simulink model "MIMO"  (R2017a)
settings: Solver=VariableStepAuto  StartTime=0.0  StopTime=inf  RelTol=1e-3
InitFcn:
  | QPSK_ini
undefined symbols (not defined in the file or in its folder): oversampling_factor, rolloff_factor
libraries: commutil2 x4, commdigbbndpm3 x4, commfilt2 x4, commsync2 x4, commrandsrc3 x2, commchan3 x2, commrflib2 x2, dspsigops x2
settings Model: Creator=Arthur  LastModifiedBy=Arthur

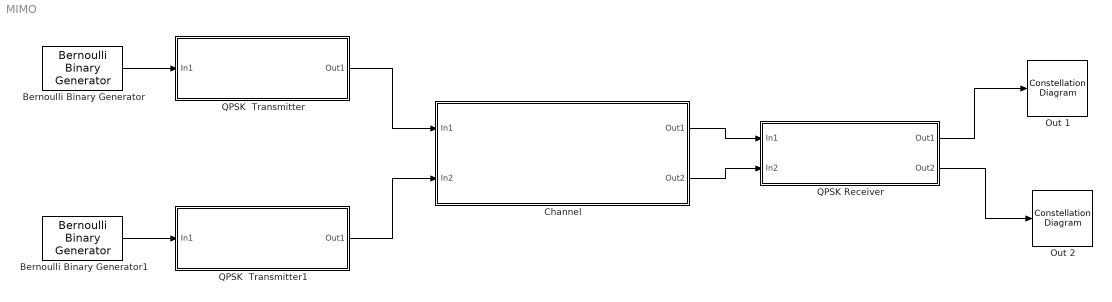
== system MIMO ==
  Bernoulli Binary Generator : commrandsrc3/Bernoulli Binary Generator  ProbabilityOfZero=0.5  SeedSource=Auto  Seed=0  SampleTime=1  SamplesPerFrame=512  OutputDataType=double  SimulateUsing=Interpreted execution
  Bernoulli Binary Generator1 : commrandsrc3/Bernoulli Binary Generator  ProbabilityOfZero=0.5  SeedSource=Auto  Seed=0  SampleTime=1  SamplesPerFrame=512  OutputDataType=double  SimulateUsing=Interpreted execution
  Channel : Subsystem
  Out 1 : ConstellationDiagram
  Out 2 : ConstellationDiagram
  QPSK  Transmitter : Subsystem
  QPSK  Transmitter1 : Subsystem
  QPSK Receiver : Subsystem
  wires:
  Bernoulli Binary Generator/1 -> QPSK  Transmitter/1(In1)
  Bernoulli Binary Generator1/1 -> QPSK  Transmitter1/1(In1)
  QPSK  Transmitter/1(Out1) -> Channel/1(In1)
  QPSK  Transmitter1/1(Out1) -> Channel/2(In2)
  Channel/1(Out1) -> QPSK Receiver/1(In1)
  QPSK Receiver/1(Out1) -> Out 1/1
  Channel/2(Out2) -> QPSK Receiver/2(In2)
  QPSK Receiver/2(Out2) -> Out 2/1

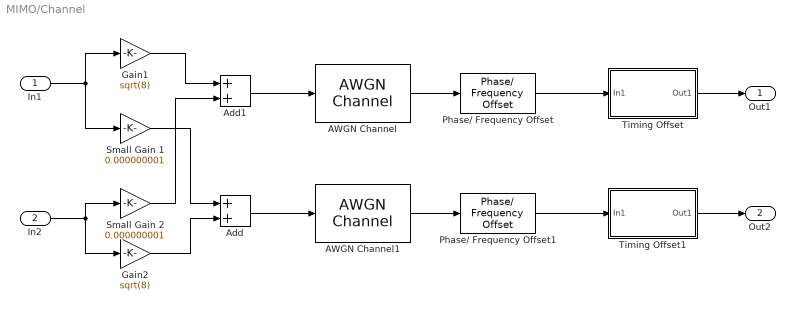
== system MIMO/Channel ==
  In1 : Inport
  In2 : Inport  Port=2
  AWGN Channel : commchan3/AWGN Channel  InputProcessing=Columns as channels (frame based)  seed=67  noiseMode="Signal to noise ratio  (Eb/No)"  EbNodB=200  EsNodB=10  SNRdB=10  bitsPerSym=2  Ps=1  Tsym=1  variance=1
  AWGN Channel1 : commchan3/AWGN Channel  InputProcessing=Columns as channels (frame based)  seed=67  noiseMode="Signal to noise ratio  (Eb/No)"  EbNodB=200  EsNodB=10  SNRdB=10  bitsPerSym=2  Ps=1  Tsym=1  variance=1
  Add : Sum
  Add1 : Sum
  Gain1 : Gain  Gain=sqrt(8)
  Gain2 : Gain  Gain=sqrt(8)
  Phase/ Frequency Offset : commrflib2/Phase// Frequency Offset  phaseOffset=0  freqPort=off  freqOffset=frequency_offset
      settings: SourceProductName=Communications System Toolbox
  Phase/ Frequency Offset1 : commrflib2/Phase// Frequency Offset  phaseOffset=0  freqPort=off  freqOffset=frequency_offset
      settings: SourceProductName=Communications System Toolbox
  Small Gain 1 : Gain  Gain=0.000000001
  Small Gain 2 : Gain  Gain=0.000000001
  Timing Offset : Subsystem
  Timing Offset1 : Subsystem
  Out1 : Outport
  Out2 : Outport  Port=2
  wires:
  AWGN Channel/1 -> Phase/ Frequency Offset/1
  In1/1 -> Small Gain 1/1, Gain1/1
  AWGN Channel1/1 -> Phase/ Frequency Offset1/1
  Phase/ Frequency Offset/1 -> Timing Offset/1(In1)
  Phase/ Frequency Offset1/1 -> Timing Offset1/1(In1)
  Timing Offset/1(Out1) -> Out1/1
  Timing Offset1/1(Out1) -> Out2/1
  Add/1 -> AWGN Channel1/1
  Small Gain 1/1 -> Add/1
  Small Gain 2/1 -> Add1/2
  Gain1/1 -> Add1/1
  Gain2/1 -> Add/2
  In2/1 -> Small Gain 2/1, Gain2/1
  Add1/1 -> AWGN Channel/1

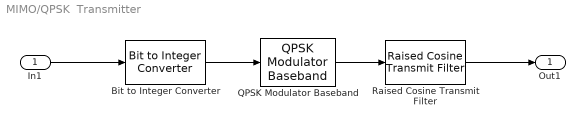
== system MIMO/QPSK  Transmitter ==
  In1 : Inport
  Bit to Integer Converter : commutil2/Bit to Integer Converter  nbits=2  bitOrder=MSB first  signedOutputValues=Unsigned  outDtype=Inherit via internal rule  outDtypeSigned=Inherit via internal rule
  QPSK Modulator Baseband : commdigbbndpm3/QPSK Modulator Baseband  InType=Integer  Enc=Gray  Ph=pi/4  outDtype=double  outWordLen=16  outUDDataType=sfix(16)  outFracLenMode=Best precision  outFracLen=15  outDataTypeStr=double  outLastDataTypeStr=double
  Raised Cosine Transmit Filter : commfilt2/Raised Cosine Transmit Filter  filtType=Square root  R=rolloff_factor  filtSpan=10  N=oversampling_factor  filterGain=1  InputProcessing=Columns as channels (frame based)  RateOptions=Enforce single-rate processing  framing=Mute  checkCoeff=off  variableName=rcTxFilt  checkGain=Normalized  sampMode=Mute  saveAsFlag=0  currentFiltSpan=10  D=5  launchFVT=on  roundingMode=Floor  overflowMode=off  coeffDataTypeStr=Inherit: Same word length as input  coeffMin=[]  coeffMax=[]  coeffLastDataTypeStr=Inherit: Same word length as input  outputDataTypeStr=Inherit: Same as accumulator  outputMin=[]  outputMax=[]  outputLastDataTypeStr=Inherit: Same as accumulator
  Out1 : Outport
  wires:
  In1/1 -> Bit to Integer Converter/1
  Bit to Integer Converter/1 -> QPSK Modulator Baseband/1
  QPSK Modulator Baseband/1 -> Raised Cosine Transmit Filter/1
  Raised Cosine Transmit Filter/1 -> Out1/1

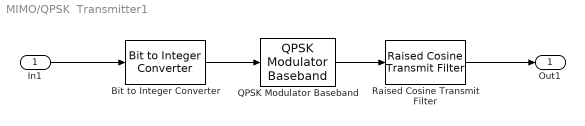
== system MIMO/QPSK  Transmitter1 ==
  In1 : Inport
  Bit to Integer Converter : commutil2/Bit to Integer Converter  nbits=2  bitOrder=MSB first  signedOutputValues=Unsigned  outDtype=Inherit via internal rule  outDtypeSigned=Inherit via internal rule
  QPSK Modulator Baseband : commdigbbndpm3/QPSK Modulator Baseband  InType=Integer  Enc=Gray  Ph=pi/4  outDtype=double  outWordLen=16  outUDDataType=sfix(16)  outFracLenMode=Best precision  outFracLen=15  outDataTypeStr=double  outLastDataTypeStr=double
  Raised Cosine Transmit Filter : commfilt2/Raised Cosine Transmit Filter  filtType=Square root  R=rolloff_factor  filtSpan=10  N=oversampling_factor  filterGain=1  InputProcessing=Columns as channels (frame based)  RateOptions=Enforce single-rate processing  framing=Mute  checkCoeff=off  variableName=rcTxFilt  checkGain=Normalized  sampMode=Mute  saveAsFlag=0  currentFiltSpan=10  D=5  launchFVT=on  roundingMode=Floor  overflowMode=off  coeffDataTypeStr=Inherit: Same word length as input  coeffMin=[]  coeffMax=[]  coeffLastDataTypeStr=Inherit: Same word length as input  outputDataTypeStr=Inherit: Same as accumulator  outputMin=[]  outputMax=[]  outputLastDataTypeStr=Inherit: Same as accumulator
  Out1 : Outport
  wires:
  In1/1 -> Bit to Integer Converter/1
  Bit to Integer Converter/1 -> QPSK Modulator Baseband/1
  QPSK Modulator Baseband/1 -> Raised Cosine Transmit Filter/1
  Raised Cosine Transmit Filter/1 -> Out1/1

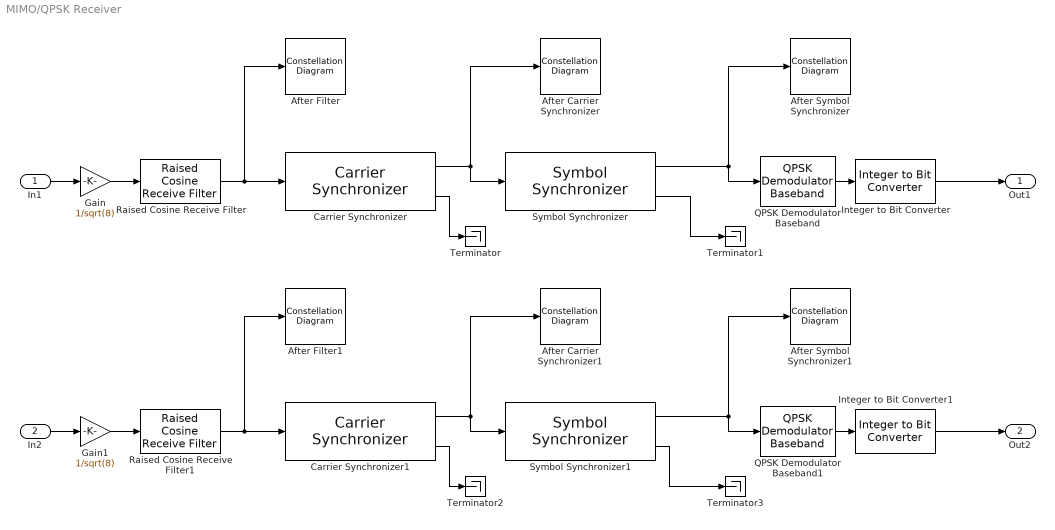
== system MIMO/QPSK Receiver ==
  In1 : Inport
  In2 : Inport  Port=2
  After Carrier Synchronizer : ConstellationDiagram
  After Carrier Synchronizer1 : ConstellationDiagram
  After Filter : ConstellationDiagram
  After Filter1 : ConstellationDiagram
  After Symbol Synchronizer : ConstellationDiagram
  After Symbol Synchronizer1 : ConstellationDiagram
  Carrier Synchronizer : commsync2/Carrier Synchronizer  Modulation=QAM  ModulationPhaseOffset=Auto  CustomPhaseOffset=0  SamplesPerSymbol=2  DampingFactor=0.707  NormalizedLoopBandwidth=0.01  EstimatedPhaseErrorOutputPort=on  SimulateUsing=Code generation
      settings: SourceProductName=Communications System Toolbox
  Carrier Synchronizer1 : commsync2/Carrier Synchronizer  Modulation=QAM  ModulationPhaseOffset=Auto  CustomPhaseOffset=0  SamplesPerSymbol=2  DampingFactor=0.707  NormalizedLoopBandwidth=0.01  EstimatedPhaseErrorOutputPort=on  SimulateUsing=Code generation
      settings: SourceProductName=Communications System Toolbox
  Gain : Gain  Gain=1/sqrt(8)
  Gain1 : Gain  Gain=1/sqrt(8)
  Integer to Bit Converter : commutil2/Integer to Bit Converter  nbits=2  signedInputValues=Unsigned  bitOrder=MSB first  outDtype=Inherit via internal rule
  Integer to Bit Converter1 : commutil2/Integer to Bit Converter  nbits=2  signedInputValues=Unsigned  bitOrder=MSB first  outDtype=Inherit via internal rule
  QPSK Demodulator Baseband : commdigbbndpm3/QPSK Demodulator Baseband  OutType=Integer  DecType=Hard decision  VarSource=Dialog  Variance=1  Dec=Gray  Ph=pi/4  outDtype1=Inherit via internal rule  outDtype2=Inherit via internal rule  derotateFactorWordLen=16  derotateFactorDataTypeStr=Inherit: Same word length as input  derotateFactorLastDataTypeStr=Inherit: Same word length as input
  QPSK Demodulator Baseband1 : commdigbbndpm3/QPSK Demodulator Baseband  OutType=Integer  DecType=Hard decision  VarSource=Dialog  Variance=1  Dec=Gray  Ph=pi/4  outDtype1=Inherit via internal rule  outDtype2=Inherit via internal rule  derotateFactorWordLen=16  derotateFactorDataTypeStr=Inherit: Same word length as input  derotateFactorLastDataTypeStr=Inherit: Same word length as input
  Raised Cosine Receive Filter : commfilt2/Raised Cosine Receive Filter  filtType=Square root  R=0.2  filtSpan=10  N=8  downFactor=1  downOffset=0  filterGain=1  InputProcessing=Columns as channels (frame based)  RateOptions=Enforce single-rate processing  framing=Mute  checkCoeff=off  variableName=rcRxFilt  currentFiltSpan=10  D=5  inputOffset=0  sampMode=Mute  saveAsFlag=0  rateMode=Downsampling  checkGain=Normalized  launchFVT=on  roundingMode=Floor  overflowMode=off  coeffDataTypeStr=Inherit: Same word length as input  coeffMin=[]  coeffMax=[]  coeffLastDataTypeStr=Inherit: Same word length as input  accumDataTypeStr=Inherit: Same as product output  accumLastDataTypeStr=Inherit: Same as product output  outputDataTypeStr=Inherit: Same as accumulator  outputMin=[]  outputMax=[]  outputLastDataTypeStr=Inherit: Same as accumulator
  Raised Cosine Receive Filter1 : commfilt2/Raised Cosine Receive Filter  filtType=Square root  R=0.2  filtSpan=10  N=8  downFactor=1  downOffset=0  filterGain=1  InputProcessing=Columns as channels (frame based)  RateOptions=Enforce single-rate processing  framing=Mute  checkCoeff=off  variableName=rcRxFilt1  currentFiltSpan=10  D=5  inputOffset=0  sampMode=Mute  saveAsFlag=0  rateMode=Downsampling  checkGain=Normalized  launchFVT=on  roundingMode=Floor  overflowMode=off  coeffDataTypeStr=Inherit: Same word length as input  coeffMin=[]  coeffMax=[]  coeffLastDataTypeStr=Inherit: Same word length as input  accumDataTypeStr=Inherit: Same as product output  accumLastDataTypeStr=Inherit: Same as product output  outputDataTypeStr=Inherit: Same as accumulator  outputMin=[]  outputMax=[]  outputLastDataTypeStr=Inherit: Same as accumulator
  Symbol Synchronizer : commsync2/Symbol Synchronizer  TimingErrorDetector=Zero-Crossing (decision-directed)  SamplesPerSymbol=8  DampingFactor=1  NormalizedLoopBandwidth=0.01  DetectorGain=2.7  TimingErrorOutputPort=on  SimulateUsing=Code generation
      settings: SourceProductName=Communications System Toolbox  SourceProductBaseCode=CM
  Symbol Synchronizer1 : commsync2/Symbol Synchronizer  TimingErrorDetector=Zero-Crossing (decision-directed)  SamplesPerSymbol=8  DampingFactor=1  NormalizedLoopBandwidth=0.01  DetectorGain=2.7  TimingErrorOutputPort=on  SimulateUsing=Code generation
      settings: SourceProductName=Communications System Toolbox  SourceProductBaseCode=CM
  Terminator{,1..3} (4 alike) : Terminator
  Out1 : Outport
  Out2 : Outport  Port=2
  wires:
  In1/1 -> Gain/1
  Raised Cosine Receive Filter/1 -> After Filter/1, Carrier Synchronizer/1
  QPSK Demodulator Baseband/1 -> Integer to Bit Converter/1
  Gain/1 -> Raised Cosine Receive Filter/1
  Integer to Bit Converter/1 -> Out1/1
  Carrier Synchronizer/1 -> Symbol Synchronizer/1, After Carrier Synchronizer/1
  Carrier Synchronizer/2 -> Terminator/1
  Symbol Synchronizer/1 -> After Symbol Synchronizer/1, QPSK Demodulator Baseband/1
  Carrier Synchronizer1/2 -> Terminator2/1
  Gain1/1 -> Raised Cosine Receive Filter1/1
  Integer to Bit Converter1/1 -> Out2/1
  Symbol Synchronizer1/1 -> After Symbol Synchronizer1/1, QPSK Demodulator Baseband1/1
  QPSK Demodulator Baseband1/1 -> Integer to Bit Converter1/1
  Symbol Synchronizer1/2 -> Terminator3/1
  Raised Cosine Receive Filter1/1 -> After Filter1/1, Carrier Synchronizer1/1
  In2/1 -> Gain1/1
  Carrier Synchronizer1/1 -> Symbol Synchronizer1/1, After Carrier Synchronizer1/1
  Symbol Synchronizer/2 -> Terminator1/1

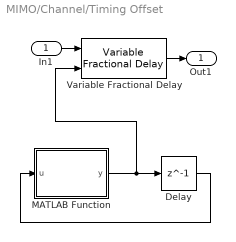
== system MIMO/Channel/Timing Offset ==
  In1 : Inport
  Delay : Delay  DelayLength=1
  MATLAB Function : MATLAB Function  TreatAsAtomicUnit=on
  Variable Fractional Delay : dspsigops/Variable Fractional Delay  mode=OBSOLETE  modeActive=Linear  dmax=30000  InputProcessing=Columns as channels (frame based)  L=4  FarrowL=4  R=10  alpha=1  ic=0  fallbackFIR=Clip to the minimum value necessary for centered kernel  fallbackFarrow=Clip to the minimum value necessary for centered kernel  noDFT=off  roundingMode=Zero  overflowMode=off
      settings: SourceProductName=DSP System Toolbox  SourceProductBaseCode=DS
  Out1 : Outport
  wires:
  Variable Fractional Delay/1 -> Out1/1
  In1/1 -> Variable Fractional Delay/1
  Delay/1 -> MATLAB Function/1(u)
  MATLAB Function/1(y) -> Variable Fractional Delay/2, Delay/1

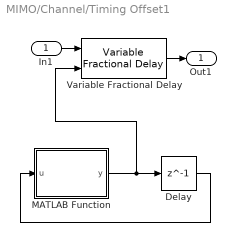
== system MIMO/Channel/Timing Offset1 ==
  In1 : Inport
  Delay : Delay  DelayLength=1
  MATLAB Function : MATLAB Function  TreatAsAtomicUnit=on
  Variable Fractional Delay : dspsigops/Variable Fractional Delay  mode=OBSOLETE  modeActive=Linear  dmax=30000  InputProcessing=Columns as channels (frame based)  L=4  FarrowL=4  R=10  alpha=1  ic=0  fallbackFIR=Clip to the minimum value necessary for centered kernel  fallbackFarrow=Clip to the minimum value necessary for centered kernel  noDFT=off  roundingMode=Zero  overflowMode=off
      settings: SourceProductName=DSP System Toolbox  SourceProductBaseCode=DS
  Out1 : Outport
  wires:
  Variable Fractional Delay/1 -> Out1/1
  In1/1 -> Variable Fractional Delay/1
  Delay/1 -> MATLAB Function/1(u)
  MATLAB Function/1(y) -> Variable Fractional Delay/2, Delay/1

== matlab function MIMO/Channel/Timing Offset1/MATLAB Function ==
  data: u input; y output
function y = fcn(u)

y = u + 0.001;

== matlab function MIMO/Channel/Timing Offset/MATLAB Function ==
  data: u input; y output
function y = fcn(u)

y = u + 0.001;
